simulink model "ReatorChernobyl"  (R2025b)
settings: Solver=VariableStepAuto  StartTime=0.0  StopTime=10.0  RelTol=1e-3
undefined symbols (not defined in the file or in its folder): beta, denG0, denGtheta, denGv, numG0, numGtheta, numGv, planta
settings Model: Creator=danilo  LastModifiedBy=danilo

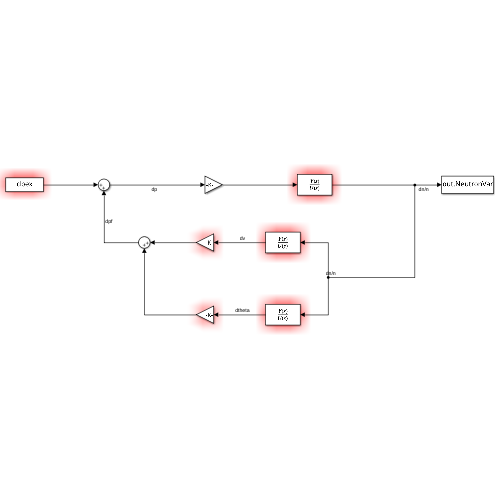
[thumbnail: Simulink's stored preview of the top-level diagram]
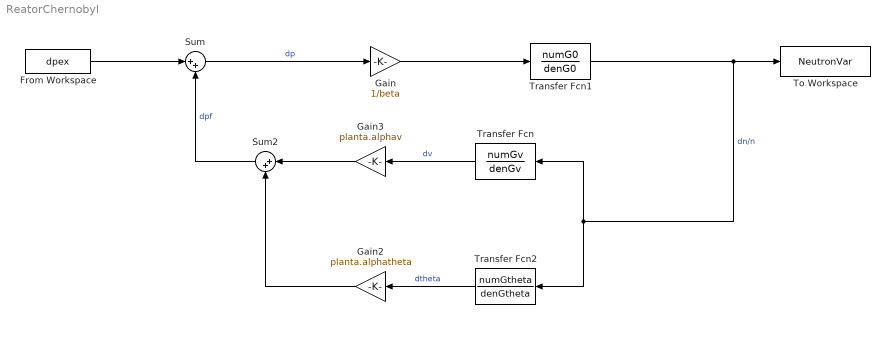
== system ReatorChernobyl ==
  From Workspace : FromWorkspace  VariableName=dpex
  Gain : Gain  Gain=1/beta
  Gain2 : Gain  Gain=planta.alphatheta
  Gain3 : Gain  Gain=planta.alphav
  Sum : Sum  Inputs=|++
  Sum2 : Sum  Inputs=|++
  To Workspace : ToWorkspace  VariableName=NeutronVar  SaveFormat=Timeseries  SampleTime=-1
  Transfer Fcn : TransferFcn  Numerator=numGv  Denominator=denGv
  Transfer Fcn1 : TransferFcn  Numerator=numG0  Denominator=denG0
  Transfer Fcn2 : TransferFcn  Numerator=numGtheta  Denominator=denGtheta
  wires:
  From Workspace/1 -> Sum/1
  Sum/1 -> Gain/1  "dp"
  Gain/1 -> Transfer Fcn1/1
  Transfer Fcn1/1 -> Transfer Fcn/1, Transfer Fcn2/1, To Workspace/1  "dn/n"
  Transfer Fcn/1 -> Gain3/1  "dv"
  Transfer Fcn2/1 -> Gain2/1  "dtheta"
  Gain3/1 -> Sum2/1
  Gain2/1 -> Sum2/2
  Sum2/1 -> Sum/2  "dpf"
